simulink model "closed_observer"  (R2024a)
settings: Solver=VariableStepAuto  StartTime=0.0  StopTime=5  MaxStep=1e-4  RelTol=1e-4
values from neighbouring files (symbols this model uses):
  A = [-40  16   9   7 ... (first row only)    [main2.m]    (also in untitled2.m = [-25 17 10 -7)
  C = [-3  2  -2  1]    [main2.m]    (also in untitled2.m = [3 -2 2 -1])
  L = L_cell{i}    [graphics.m]
  x0 = [1 1 1 1]'    [main2.m]    (also in untitled2.m)
  x0_hat = [0 0 0 0]'    [main2.m]    (also in untitled2.m)
settings Model: Creator=eva  LastModifiedBy=eva

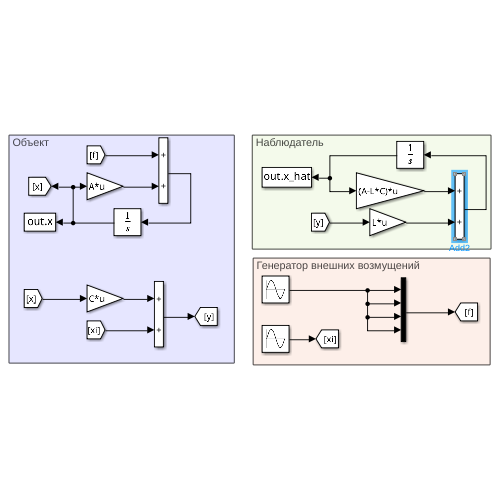
[thumbnail: Simulink's stored preview of the top-level diagram]
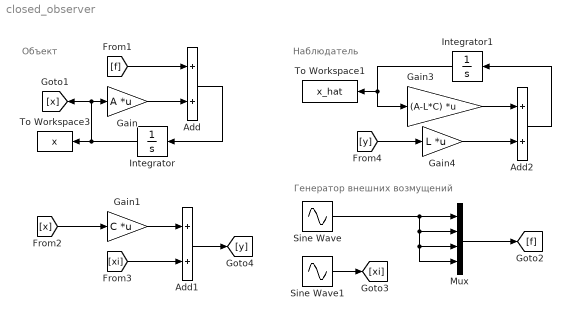
== system closed_observer ==
  note: Наблюдатель
  note: Генератор внешних возмущений
  note: Объект
  Add : Sum
  Add1 : Sum
  Add2 : Sum
  Gain : Gain  Gain=A  Multiplication=Matrix(K*u)
  Gain1 : Gain  Gain=C  Multiplication=Matrix(K*u)
  Gain3 : Gain  Gain=(A-L*C)  Multiplication=Matrix(K*u)
  Gain4 : Gain  Gain=L  Multiplication=Matrix(K*u)
  Integrator : Integrator  InitialCondition=x0
  Integrator1 : Integrator  InitialCondition=x0_hat
  Mux : Mux
  Sine Wave : Sin  Amplitude=0.5  Frequency=2  SampleTime=0
  Sine Wave1 : Sin  Amplitude=0.1  Frequency=5  Phase=pi/4  SampleTime=0
  To Workspace1 : ToWorkspace  VariableName=x_hat  SaveFormat=Structure With Time  SampleTime=-1
  To Workspace3 : ToWorkspace  VariableName=x  SaveFormat=Structure With Time  SampleTime=-1
  wires:
  [f] -> Add/1
  Sine Wave/1 -> Mux/1, Mux/3, Mux/4, Mux/2
  Mux/1 -> [f]
  Sine Wave1/1 -> [xi]
  Gain/1 -> Add/2
  Add/1 -> Integrator/1
  [x] -> Gain1/1
  Gain1/1 -> Add1/1
  [xi] -> Add1/2
  Add1/1 -> [y]
  Integrator/1 -> To Workspace3/1, [x], Gain/1
  [y] -> Gain4/1
  Gain4/1 -> Add2/2
  Gain3/1 -> Add2/1
  Add2/1 -> Integrator1/1
  Integrator1/1 -> To Workspace1/1, Gain3/1
